simulink model "bai_huong_dan_day_3"  (R2024a)
settings: Solver=FixedStepAuto  StartTime=0.0  StopTime=10.0  FixedStep=0.1  RelTol=1e-3
undefined symbols (not defined in the file): Sheet1
libraries: simulink x7
settings Model: Creator=user  LastModifiedBy=user
settings OptimizationCC: DefaultParameterBehavior=Inlined  EnhancedBackFolding=on  PassReuseOutputArgsAs=Individual arguments  ZeroExternalMemoryAtStartup=off  ZeroInternalMemoryAtStartup=off  OptimizeBlockOrder=speed  DifferentSizesBufferReuse=on  OptimizationCustomize=off  EfficientTunableParamExpr=on
settings DebuggingCC: ParameterTunabilityLossMsg=error
settings SFSimCC: MATLABDynamicMemAlloc=off
settings RTWCC: Description=Embedded Coder  SystemTargetFile=ert.tlc  TemplateMakefile=ert_default_tmf
settings CodeAppCC: ForceParamTrailComments=on  IgnoreCustomStorageClasses=off  OperatorAnnotations=on  SimulinkDataObjDesc=on  SFDataObjDesc=on  InsertBlockDesc=on
settings ERTTargetCC: TargetLangStandard=C99 (ISO)  GenerateSampleERTMain=on  InlinedParameterPlacement=NonHierarchical  ERTCustomFileTemplate=example_file_process.tlc

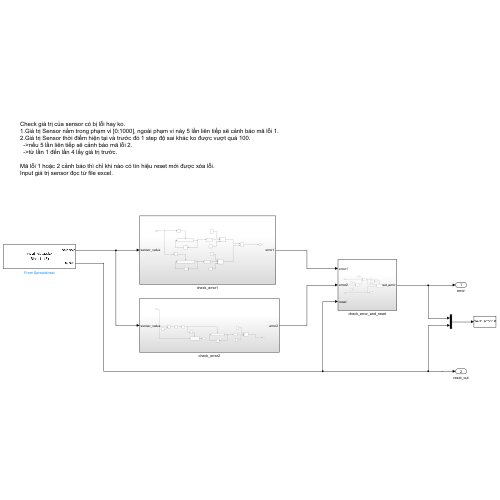
[thumbnail: Simulink's stored preview of the top-level diagram]
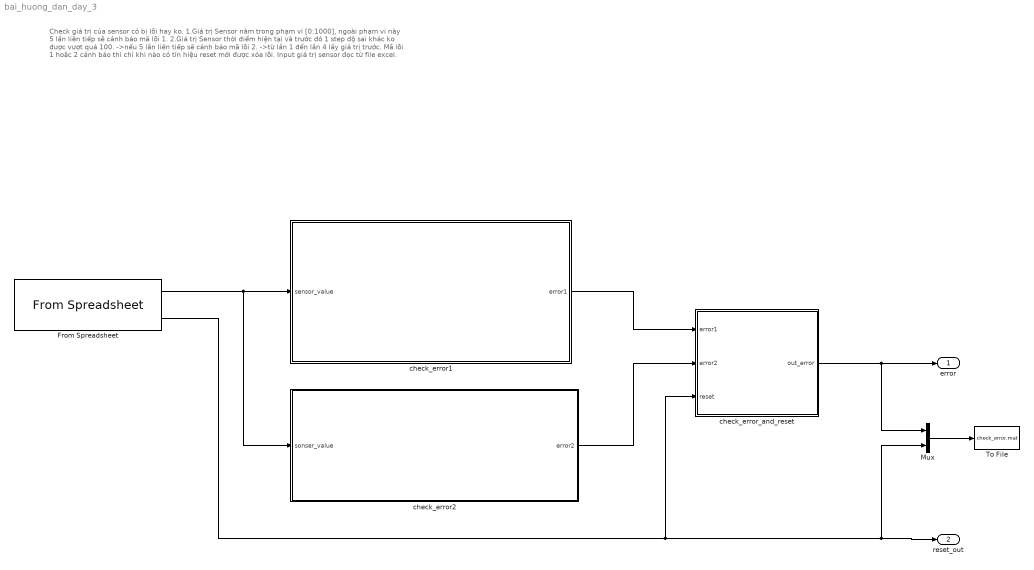
== system bai_huong_dan_day_3 ==
  note: Check giá trị của sensor có bị lỗi hay ko.
      | 1.Giá trị Sensor nằm trong phạm vi [0:1000], ngoài phạm vi này 5 lần liên tiếp sẽ cảnh báo mã lỗi 1.
      | 2.Giá trị Sensor thời điểm hiện tại và trước đó 1 step độ sai khác ko được vượt quá 100.
      |   ->nếu 5 lần liên tiếp sẽ cảnh báo mã lỗi 2.
      |   ->từ lần 1 đến lần 4 lấy giá trị trước.
      |
      | Mã lỗi 1 hoặc 2 cảnh báo thì chỉ khi nào có tín hiệu reset mới được xóa lỗi.
      | Input giá trị sensor đọc từ file excel.
  From Spreadsheet : FromSpreadsheet  FileName=input_data.xlsx  SheetName=Sheet1 (2)
  Mux : Mux  Inputs=2
  To File : ToFile  Filename=check_error.mat  SaveFormat=Timeseries
  check_error1 : Subsystem
  check_error2 : Subsystem
  check_error_and_reset : Subsystem
  error : Outport
  reset_out : Outport  Port=2
  wires:
  From Spreadsheet/1 -> check_error2/1(sonser_value), check_error1/1(sensor_value)
  check_error1/1(error1) -> check_error_and_reset/1(error1)
  check_error2/1(error2) -> check_error_and_reset/2(error2)
  check_error_and_reset/1(out_error) -> Mux/1, error/1
  From Spreadsheet/2 -> Mux/2, reset_out/1, check_error_and_reset/3(reset)
  Mux/1 -> To File/1

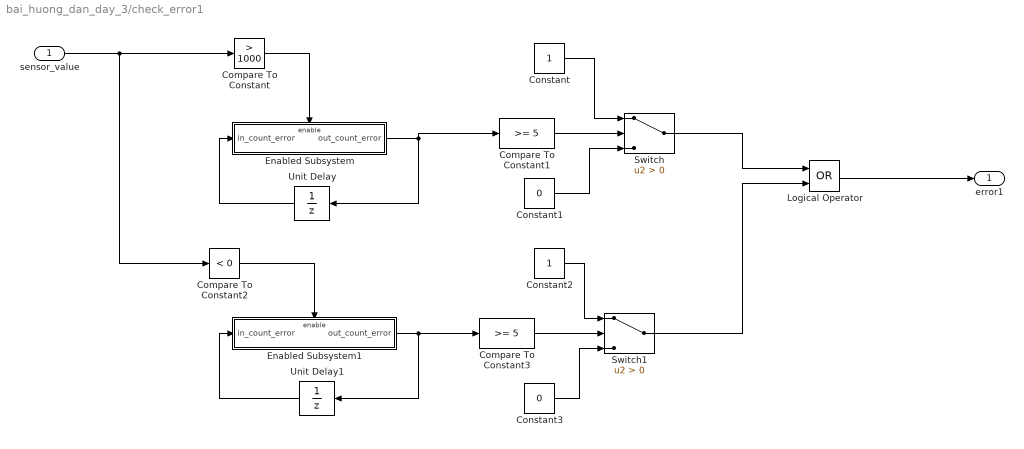
== system bai_huong_dan_day_3/check_error1 ==
  sensor_value : Inport
  Compare To Constant : simulink/Logic and Bit Operations/Compare To Constant  relop=>  const=1000  OutDataTypeStr=boolean
  Compare To Constant1 : simulink/Logic and Bit Operations/Compare To Constant  relop=>=  const=5  OutDataTypeStr=boolean
  Compare To Constant2 : simulink/Logic and Bit Operations/Compare To Constant  relop=<  const=0  OutDataTypeStr=boolean
  Compare To Constant3 : simulink/Logic and Bit Operations/Compare To Constant  relop=>=  const=5  OutDataTypeStr=boolean
  Constant : Constant
  Constant1 : Constant  Value=0
  Constant2 : Constant
  Constant3 : Constant  Value=0
  Enabled Subsystem : Subsystem  TreatAsAtomicUnit=on
  Enabled Subsystem1 : Subsystem  TreatAsAtomicUnit=on
  Logical Operator : Logic  Operator=OR  AllPortsSameDT=off  OutDataTypeStr=boolean
  Switch : Switch  Criteria=u2 > Threshold  SaturateOnIntegerOverflow=off  InputSameDT=off
  Switch1 : Switch  Criteria=u2 > Threshold  SaturateOnIntegerOverflow=off  InputSameDT=off
  Unit Delay : UnitDelay  SampleTime=-1  HasFrameUpgradeWarning=on
  Unit Delay1 : UnitDelay  SampleTime=-1  HasFrameUpgradeWarning=on
  error1 : Outport
  wires:
  Constant/1 -> Switch/1
  Constant2/1 -> Switch1/1
  Unit Delay/1 -> Enabled Subsystem/1(in_count_error)
  Compare To Constant/1 -> Enabled Subsystem/Enable
  sensor_value/1 -> Compare To Constant/1, Compare To Constant2/1
  Enabled Subsystem/1(out_count_error) -> Compare To Constant1/1, Unit Delay/1
  Compare To Constant1/1 -> Switch/2
  Constant3/1 -> Switch1/3
  Switch/1 -> Logical Operator/1
  Enabled Subsystem1/1(out_count_error) -> Unit Delay1/1, Compare To Constant3/1
  Unit Delay1/1 -> Enabled Subsystem1/1(in_count_error)
  Logical Operator/1 -> error1/1
  Compare To Constant3/1 -> Switch1/2
  Compare To Constant2/1 -> Enabled Subsystem1/Enable
  Switch1/1 -> Logical Operator/2
  Constant1/1 -> Switch/3

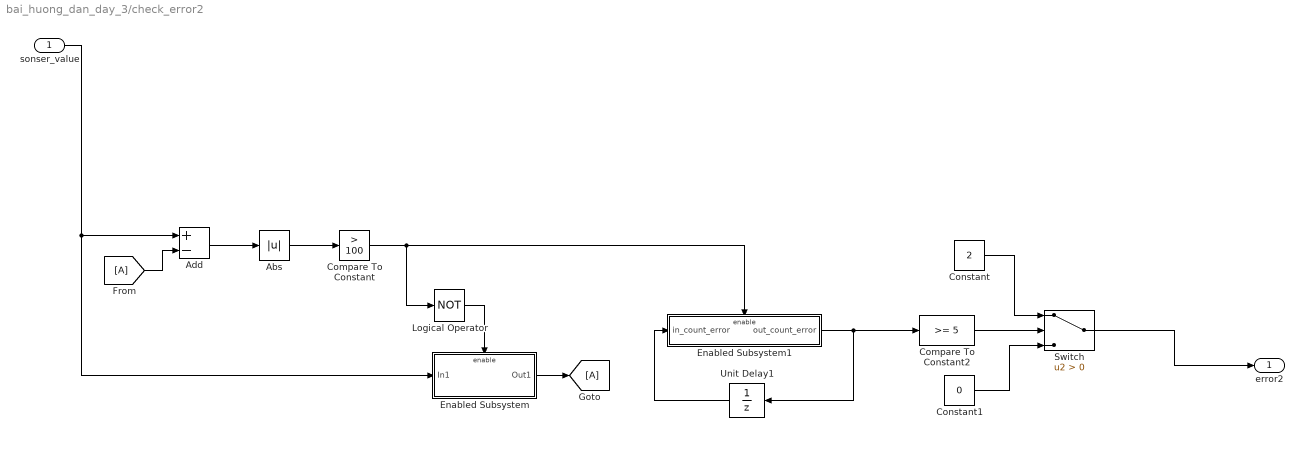
== system bai_huong_dan_day_3/check_error2 ==
  sonser_value : Inport
  Abs : Abs  SaturateOnIntegerOverflow=off
  Add : Sum  Inputs=+-
  Compare To Constant : simulink/Logic and Bit Operations/Compare To Constant  relop=>  const=100  OutDataTypeStr=boolean
  Compare To Constant2 : simulink/Logic and Bit Operations/Compare To Constant  relop=>=  const=5  OutDataTypeStr=boolean
  Constant : Constant  Value=2
  Constant1 : Constant  Value=0
  Enabled Subsystem : Subsystem  TreatAsAtomicUnit=on
  Enabled Subsystem1 : Subsystem  TreatAsAtomicUnit=on
  From : From
  Goto : Goto
  Logical Operator : Logic  Operator=NOT  AllPortsSameDT=off  OutDataTypeStr=boolean
  Switch : Switch  Criteria=u2 > Threshold  SaturateOnIntegerOverflow=off  InputSameDT=off
  Unit Delay1 : UnitDelay  SampleTime=-1  HasFrameUpgradeWarning=on
  error2 : Outport
  wires:
  Add/1 -> Abs/1
  Enabled Subsystem1/1(out_count_error) -> Unit Delay1/1, Compare To Constant2/1
  From/1 -> Add/2
  Constant1/1 -> Switch/3
  Enabled Subsystem/1(Out1) -> Goto/1
  Compare To Constant/1 -> Enabled Subsystem1/Enable, Logical Operator/1
  Abs/1 -> Compare To Constant/1
  sonser_value/1 -> Enabled Subsystem/1(In1), Add/1
  Logical Operator/1 -> Enabled Subsystem/Enable
  Unit Delay1/1 -> Enabled Subsystem1/1(in_count_error)
  Compare To Constant2/1 -> Switch/2
  Constant/1 -> Switch/1
  Switch/1 -> error2/1

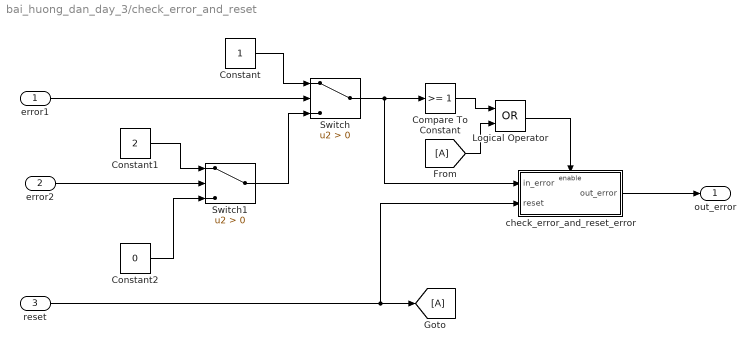
== system bai_huong_dan_day_3/check_error_and_reset ==
  error1 : Inport
  error2 : Inport  Port=2
  reset : Inport  Port=3
  Compare To Constant : simulink/Logic and Bit Operations/Compare To Constant  relop=>=  const=1  OutDataTypeStr=boolean
  Constant : Constant
  Constant1 : Constant  Value=2
  Constant2 : Constant  Value=0
  From : From
  Goto : Goto
  Logical Operator : Logic  Operator=OR  AllPortsSameDT=off  OutDataTypeStr=boolean
  Switch : Switch  Criteria=u2 > Threshold  SaturateOnIntegerOverflow=off  InputSameDT=off
  Switch1 : Switch  Criteria=u2 > Threshold  SaturateOnIntegerOverflow=off  InputSameDT=off
  check_error_and_reset_error : Subsystem  TreatAsAtomicUnit=on
  out_error : Outport
  wires:
  Constant/1 -> Switch/1
  Compare To Constant/1 -> Logical Operator/1
  reset/1 -> Goto/1, check_error_and_reset_error/2(reset)
  Switch1/1 -> Switch/3
  Switch/1 -> check_error_and_reset_error/1(in_error), Compare To Constant/1
  Constant2/1 -> Switch1/3
  Logical Operator/1 -> check_error_and_reset_error/Enable
  Constant1/1 -> Switch1/1
  From/1 -> Logical Operator/2
  error2/1 -> Switch1/2
  error1/1 -> Switch/2
  check_error_and_reset_error/1(out_error) -> out_error/1

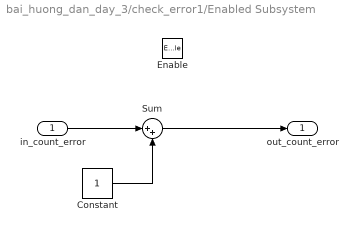
== system bai_huong_dan_day_3/check_error1/Enabled Subsystem ==
  in_count_error : Inport
  Enable : EnablePort  StatesWhenEnabling=reset
  Constant : Constant
  Sum : Sum  Inputs=|++
  out_count_error : Outport  OutputWhenDisabled=reset  InitialOutput=0
  wires:
  in_count_error/1 -> Sum/1
  Constant/1 -> Sum/2
  Sum/1 -> out_count_error/1

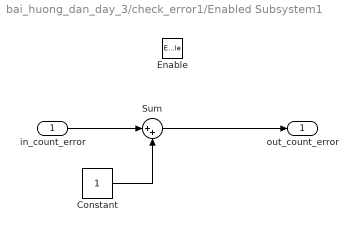
== system bai_huong_dan_day_3/check_error1/Enabled Subsystem1 ==
  in_count_error : Inport
  Enable : EnablePort  StatesWhenEnabling=reset
  Constant : Constant
  Sum : Sum  Inputs=|++
  out_count_error : Outport  OutputWhenDisabled=reset  InitialOutput=0
  wires:
  in_count_error/1 -> Sum/1
  Constant/1 -> Sum/2
  Sum/1 -> out_count_error/1

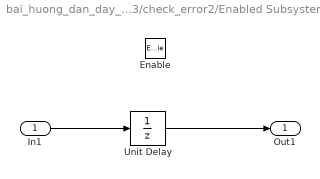
== system bai_huong_dan_day_3/check_error2/Enabled Subsystem ==
  In1 : Inport
  Enable : EnablePort
  Unit Delay : UnitDelay  SampleTime=-1  HasFrameUpgradeWarning=on
  Out1 : Outport
  wires:
  In1/1 -> Unit Delay/1
  Unit Delay/1 -> Out1/1

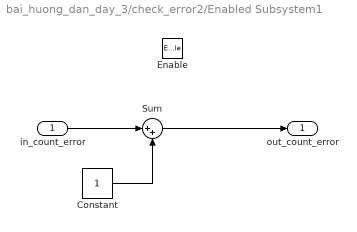
== system bai_huong_dan_day_3/check_error2/Enabled Subsystem1 ==
  in_count_error : Inport
  Enable : EnablePort  StatesWhenEnabling=reset
  Constant : Constant
  Sum : Sum  Inputs=|++
  out_count_error : Outport  OutputWhenDisabled=reset  InitialOutput=0
  wires:
  in_count_error/1 -> Sum/1
  Constant/1 -> Sum/2
  Sum/1 -> out_count_error/1

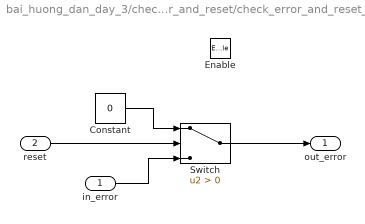
== system bai_huong_dan_day_3/check_error_and_reset/check_error_and_reset_error ==
  in_error : Inport
  reset : Inport  Port=2
  Enable : EnablePort
  Constant : Constant  Value=0
  Switch : Switch  Criteria=u2 > Threshold  SaturateOnIntegerOverflow=off  InputSameDT=off
  out_error : Outport
  wires:
  reset/1 -> Switch/2
  Constant/1 -> Switch/1
  in_error/1 -> Switch/3
  Switch/1 -> out_error/1
